simulink model "Maxon_MSM_Motor_Step_Response"  (R2015a)
settings: Solver=ode3  SolverMode=SingleTasking  StartTime=0.0  StopTime=inf  FixedStep=.005  RelTol=1e-3
libraries: RASPlib x3, MinSegLibrary_MinSegMega x2
settings Model: ExtModeTrigDuration=2  Creator=malcoj2  LastModifiedBy=hurstj
settings OptimizationCC: OptimizeModelRefInitCode=on  LifeSpan=1
settings DebuggingCC: UnderspecifiedInitializationDetection=Classic  MergeDetectMultiDrivingBlocksExec=none  StateNameClashWarn=warning
settings HardwareCC: ProdBitPerInt=16  ProdBitPerPointer=8  ProdIntDivRoundTo=Zero  ProdEndianess=LittleEndian  ProdWordSize=8  ProdHWDeviceType=Atmel->AVR
settings RTWCC: SystemTargetFile=realtime.tlc  GenerateMakefile=off  TemplateMakefile=realtime.tmf  Description=Run on Target Hardware  RTWVerbose=off
settings ERTTargetCC: CombineOutputUpdateFcns=off  ExtModeTransport=3  ExtModeMexFile=ext_serial_win32_comm_rtt  ExtModeMexArgs=0 1 9600  ERTSrcFileBannerTemplate=realtime_code_template.cgt  ERTHdrFileBannerTemplate=realtime_code_template.cgt  ERTDataSrcFileTemplate=realtime_code_template.cgt  ERTDataHdrFileTemplate=realtime_code_template.cgt  ERTCustomFileTemplate=realtime_file_process.tlc

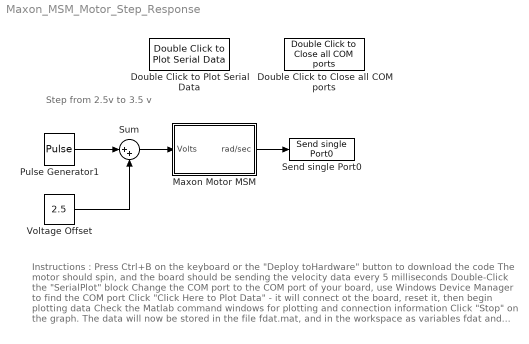
== system Maxon_MSM_Motor_Step_Response ==
  note: Step from 2.5v
      | to 3.5 v
  note: Instructions :
      | Press Ctrl+B on the keyboard or the "Deploy toHardware" button to download the code
      | The motor should spin, and the board should be sending the velocity data every 5 milliseconds
      | Double-Click the "SerialPlot" block
      | Change the COM port to the COM port of your board, use Windows Device Manager to find the COM port
      | Click "Click Here to Plot Data" - it will connect ot the board, reset it, then begin plotting data
      | Check the Matlab command windows for plotting and connection information
      | Click "Stop" on the graph. The data will now be stored in the file fdat.mat, and in the workspace as variables fdat and wdat
      | Plot the data by typing "plot(fdat)" in the MATLAB command window
      | Rename the file "fdat.mat" in the current folder to a meaninful name to ensure you keep the data
      |
      | The sample time can be modified in the in the "Configuration Parameters" which can be accessed by the wheel in the toolbar, right clicking on the simulation diagram of pressing Ctrl+E on the keyboard
  Double Click to Close all COM ports : RASPlib/Double Click to Close all COM ports
  Double Click to Plot Serial Data : RASPlib/Double Click to Plot Serial Data  COMport=127  BaudRate=9600  NumSamples=500  DataType=single
  Maxon Motor MSM : Subsystem
  Pulse Generator1 : DiscretePulseGenerator  PulseType=Time based  Period=8  PulseWidth=50
  Send single Port0 : RASPlib/Send single Port0
  Sum : Sum  Inputs=|++
  Voltage Offset : Constant  Value=2.5
  wires:
  Maxon Motor MSM/1(rad/sec) -> Send single Port0/1
  Pulse Generator1/1 -> Sum/1
  Voltage Offset/1 -> Sum/2
  Sum/1 -> Maxon Motor MSM/1(Volts)

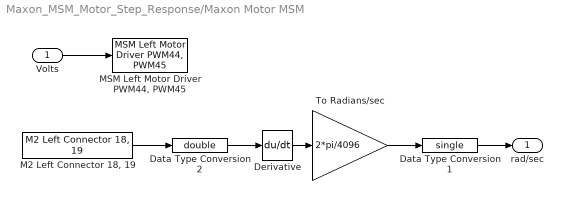
== system Maxon_MSM_Motor_Step_Response/Maxon Motor MSM ==
  Volts : Inport
  Data Type Conversion1 : DataTypeConversion  OutDataTypeStr=single
  Data Type Conversion2 : DataTypeConversion  OutDataTypeStr=double
  Derivative : Derivative
  "M2 Left Connector 18, 19" : MinSegLibrary_MinSegMega/M2 Left Connector 18, 19  Encoder=1  PinA=19  PinB=18  PWMFSelect=3  PWMTimer=-1
  "MSM Left Motor Driver PWM44, PWM45" : MinSegLibrary_MinSegMega/MSM Left Motor Driver PWM44, PWM45  Vsupply=3.9  PWMoffset=0
  To Radians/sec : Gain  Gain=2*pi/4096
  rad/sec : Outport
  wires:
  Derivative/1 -> To Radians/sec/1
  Volts/1 -> "MSM Left Motor Driver PWM44, PWM45"/1
  To Radians/sec/1 -> Data Type Conversion1/1
  "M2 Left Connector 18, 19"/1 -> Data Type Conversion2/1
  Data Type Conversion2/1 -> Derivative/1
  Data Type Conversion1/1 -> rad/sec/1
